simulink model "Model_eCVT"  (R2019a)
settings: Solver=ode45  StartTime=0.0  StopTime=5  RelTol=1e-3
undefined symbols (not defined in the file): alpha, Be, Je, Kd, Ki, Kp, Kpot, Kpwm, Kspring, Kt, Kv, La, r, Ra, tau, Ts
libraries: simulink x3
settings Model: Creator=Safet  LastModifiedBy=Safet
settings SolverCC: ZeroCrossAlgorithm=Adaptive
settings DebuggingCC: IgnoredZcDiagnostic=none

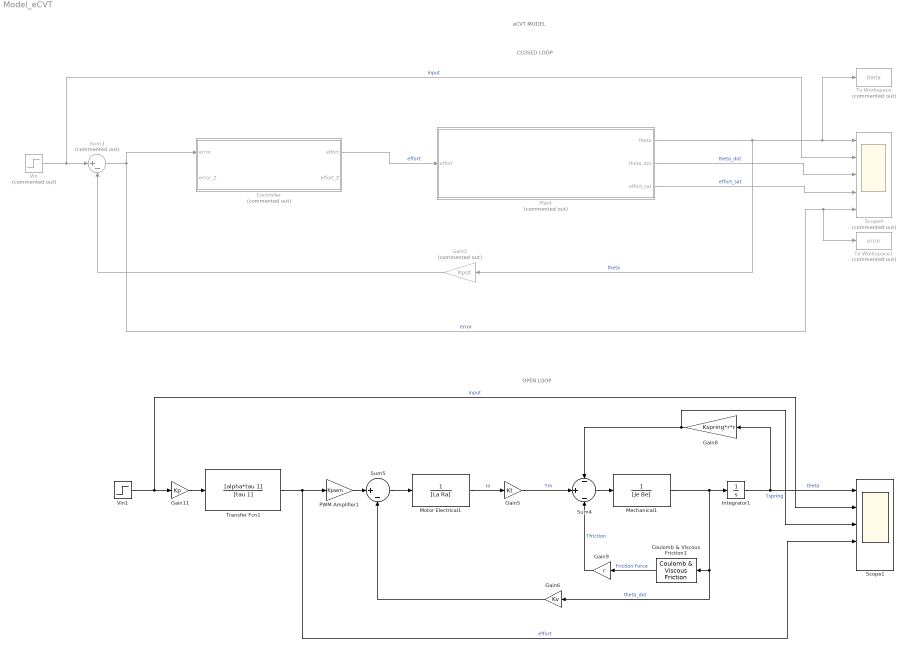
== system Model_eCVT ==
  note: OPEN LOOP
  note: eCVT MODEL
  note: CLOSED LOOP
  Controller : Subsystem  Commented=on
  Coulomb & Viscous Friction1 : simulink/Discontinuities/Coulomb & Viscous Friction  offset=0.2  gain=Be
      settings: SourceProductName=Simulink
  Gain11 : Gain  Gain=Kp
  Gain2 : Gain  Commented=on  Gain=Kpot
  Gain5 : Gain  Gain=Kt
  Gain6 : Gain  Gain=Kv
  Gain8 : Gain  Gain=Kspring*r*r
  Gain9 : Gain  Gain=r
  Integrator1 : Integrator
  Mechanical1 : TransferFcn  Denominator=[Je Be]
  Motor Electrical1 : TransferFcn  Denominator=[La Ra]
  PWM Amplifier1 : Gain  Gain=Kpwm
  Plant : Subsystem  Commented=on
  Scope1 : Scope  NumInputPorts=5
  Scope4 : Scope  Commented=on  NumInputPorts=5
  Sum3 : Sum  Commented=on  Inputs=|+-
  Sum4 : Sum  Inputs=-|+|-
  Sum5 : Sum  Inputs=|+-
  To Workspace : ToWorkspace  Commented=on  VariableName=theta  SaveFormat=Timeseries  SampleTime=-1
  To Workspace1 : ToWorkspace  Commented=on  VariableName=error  SaveFormat=Timeseries  SampleTime=-1
  Transfer Fcn1 : TransferFcn  Numerator=[alpha*tau 1]  Denominator=[tau 1]
  Vin : Step  Commented=on  Time=0  After=1.0612  SampleTime=0
  Vin1 : Step  After=1.06  SampleTime=0
  wires:
  Sum3/1 -> Controller/1(error), To Workspace1/1, Scope4/5  "error"
  Vin/1 -> Scope4/2, Sum3/1  "input"
  Gain2/1 -> Sum3/2
  Motor Electrical1/1 -> Gain5/1  "Ia"
  Sum4/1 -> Mechanical1/1
  Mechanical1/1 -> Coulomb & Viscous Friction1/1, Gain6/1, Integrator1/1  "theta_dot"
  Gain8/1 -> Sum4/1, Scope1/3  "Tspring"
  Gain5/1 -> Sum4/2  "Tm"
  Sum5/1 -> Motor Electrical1/1
  PWM Amplifier1/1 -> Sum5/1
  Integrator1/1 -> Gain8/1, Scope1/1  "theta"
  Vin1/1 -> Scope1/2, Gain11/1  "input"
  Gain9/1 -> Sum4/3  "Tfriction"
  Gain6/1 -> Sum5/2
  Coulomb & Viscous Friction1/1 -> Gain9/1  "Friction Force"
  Transfer Fcn1/1 -> Scope1/4, PWM Amplifier1/1  "effort"
  Gain11/1 -> Transfer Fcn1/1
  Plant/1(theta) -> To Workspace/1, Scope4/1, Gain2/1  "theta"
  Plant/2("theta_dot ") -> Scope4/3  "theta_dot"
  Plant/3("effort_sat ") -> Scope4/4  "effort_sat"
  Controller/1(effort) -> Plant/1("effort ")  "effort"

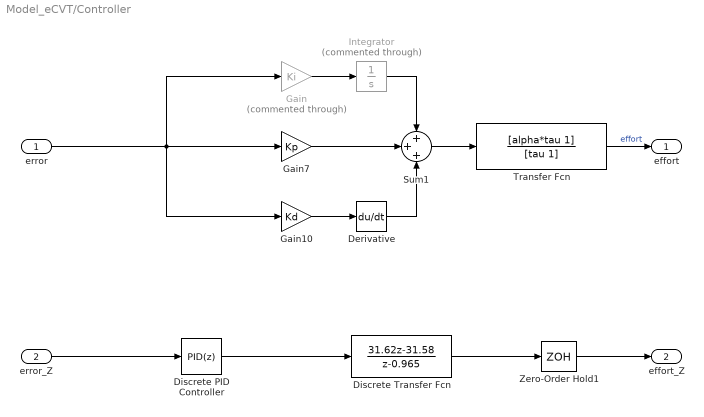
== system Model_eCVT/Controller ==
  error : Inport
  error_Z : Inport  Port=2
  Derivative : Derivative
  Discrete Transfer Fcn : DiscreteTransferFcn  Numerator=[31.62 -31.58]  Denominator=[1 -0.965]
  Discrete PID Controller : simulink/Continuous/PID Controller  Controller=PID  Form=Parallel  TimeDomain=Discrete-time  SampleTime=-1  IntegratorMethod=Forward Euler  FilterMethod=Forward Euler  ControllerParametersSource=internal  P=Kp  I=Ki  D=Kd  UseFilter=on  N=100  TunerSelectOption=Transfer Function Based (PID Tuner App)  InitialConditionSource=internal  InitialConditionForIntegrator=0  InitialConditionForFilter=0  DifferentiatorICPrevScaledInput=0  ExternalReset=none  TrackingMode=off  Kt=1  LimitOutput=off  UpperSaturationLimit=inf  LowerSaturationLimit=-inf  LinearizeAsGain=off  AntiWindupMode=none  Kb=1  POutMin=[]  POutMax=[]  IOutMin=[]  IOutMax=[]  DOutMin=[]  DOutMax=[]  NOutMin=[]  NOutMax=[]  SumOutMin=[]  SumOutMax=[]  SaturationOutMin=[]  SaturationOutMax=[]  PParamMin=[]  PParamMax=[]  IParamMin=[]  IParamMax=[]  DParamMin=[]  DParamMax=[]  NParamMin=[]  NParamMax=[]  KbParamMin=[]  KbParamMax=[]  KtParamMin=[]  KtParamMax=[]  KbOutMin=[]  KbOutMax=[]  KtOutMin=[]  KtOutMax=[]  IntegratorOutMin=[]  IntegratorOutMax=[]  FilterOutMin=[]  FilterOutMax=[]  SumI1OutMin=[]  SumI1OutMax=[]  SumI2OutMin=[]  SumI2OutMax=[]  SumI3OutMin=[]  SumI3OutMax=[]  SumI4OutMin=[]  SumI4OutMax=[]  SumDOutMin=[]  SumDOutMax=[]  DifferentiatorOutMin=[]  DifferentiatorOutMax=[]  FilterDiffOutCoefMin=[]  FilterDiffOutCoefMax=[]  ReciprocalOutMin=[]  ReciprocalOutMax=[]  SumDenOutMin=[]  SumDenOutMax=[]  SumNumOutMin=[]  SumNumOutMax=[]  DivideOutMin=[]  DivideOutMax=[]  IntegratorContinuousStateAttributes=''  IntegratorStateMustResolveToSignalObject=off  IntegratorRTWStateStorageClass=Auto  FilterContinuousStateAttributes=''  FilterStateMustResolveToSignalObject=off  FilterRTWStateStorageClass=Auto  ParallelPVariant=InternalParameters  IdealPVariant=Disabled  IVariant=InternalParameters  DVariant=InternalParameters  IntegratorVariant=Discrete  SatVariant=Disabled  AWVariant=Passthrough  PCopyVariant=Disabled  TRVariant=Disabled  FdbkBlocksVariant=Forward  IdealPFdbkVariant=Disabled  SatFdbkVariant=Disabled  DerivativeFilterVariant=ForwardEulerFilter  NVariant=InternalParameters  NCopyVariant=Disabled  FilterICVariant=InternalICsFilter  IntegratorICVariant=InternalICs  ExternalResetVariant=Disabled  TRSumVariant=Passthrough  SumFdbkVariant=Disabled  SumVariant=Sum_PID
  Gain : Gain  Commented=through  Gain=Ki
  Gain10 : Gain  Gain=Kd
  Gain7 : Gain  Gain=Kp
  Integrator : Integrator  Commented=through
  Sum1 : Sum  Inputs=+++
  Transfer Fcn : TransferFcn  Numerator=[alpha*tau 1]  Denominator=[tau 1]
  Zero-Order Hold1 : ZeroOrderHold  SampleTime=Ts
  effort : Outport
  effort_Z : Outport  Port=2
  wires:
  Derivative/1 -> Sum1/3
  Sum1/1 -> Transfer Fcn/1
  Transfer Fcn/1 -> effort/1  "effort"
  Gain7/1 -> Sum1/2
  Gain10/1 -> Derivative/1
  error/1 -> Gain/1, Gain10/1, Gain7/1
  Gain/1 -> Integrator/1
  Integrator/1 -> Sum1/1
  Discrete Transfer Fcn/1 -> Zero-Order Hold1/1
  Zero-Order Hold1/1 -> effort_Z/1
  Discrete PID Controller/1 -> Discrete Transfer Fcn/1
  error_Z/1 -> Discrete PID Controller/1

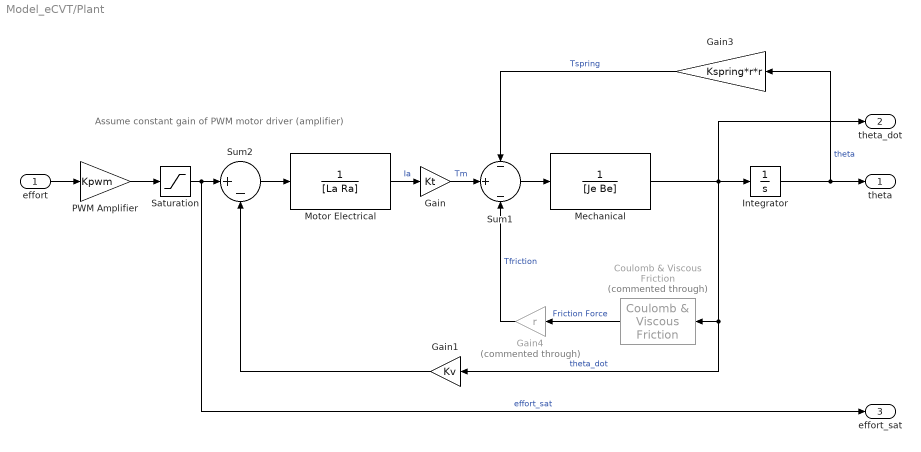
== system Model_eCVT/Plant ==
  note: Assume constant gain of PWM motor driver (amplifier)
  "effort " : Inport
  Coulomb & Viscous Friction : simulink/Discontinuities/Coulomb & Viscous Friction  Commented=through  offset=0.2  gain=Be
      settings: SourceProductName=Simulink
  Gain : Gain  Gain=Kt
  Gain1 : Gain  Gain=Kv
  Gain3 : Gain  Gain=Kspring*r*r
  Gain4 : Gain  Commented=through  Gain=r
  Integrator : Integrator
  Mechanical : TransferFcn  Denominator=[Je Be]
  Motor Electrical : TransferFcn  Denominator=[La Ra]
  PWM Amplifier : Gain  Gain=Kpwm
  Saturation : Saturate  UpperLimit=6  LowerLimit=-6
  Sum1 : Sum  Inputs=-|+|-
  Sum2 : Sum  Inputs=|+-
  theta : Outport
  "theta_dot " : Outport  Port=2
  "effort_sat " : Outport  Port=3
  wires:
  Motor Electrical/1 -> Gain/1  "Ia"
  Gain4/1 -> Sum1/3  "Tfriction"
  Coulomb & Viscous Friction/1 -> Gain4/1  "Friction Force"
  "effort "/1 -> PWM Amplifier/1
  Mechanical/1 -> "theta_dot "/1, Integrator/1, Coulomb & Viscous Friction/1, Gain1/1  "theta_dot"
  Gain1/1 -> Sum2/2
  Gain/1 -> Sum1/2  "Tm"
  Gain3/1 -> Sum1/1  "Tspring"
  Sum1/1 -> Mechanical/1
  PWM Amplifier/1 -> Saturation/1
  Sum2/1 -> Motor Electrical/1
  Integrator/1 -> Gain3/1, theta/1  "theta"
  Saturation/1 -> "effort_sat "/1, Sum2/1  "effort_sat"
